simulink model "sampleModel1660"  (R2023a)
settings: Solver=VariableStepAuto  StartTime=0.0  StopTime=10.0  RelTol=1e-3
libraries: hdlsllib x7, simulink x4
settings Model: Creator=user1  LastModifiedBy=user1

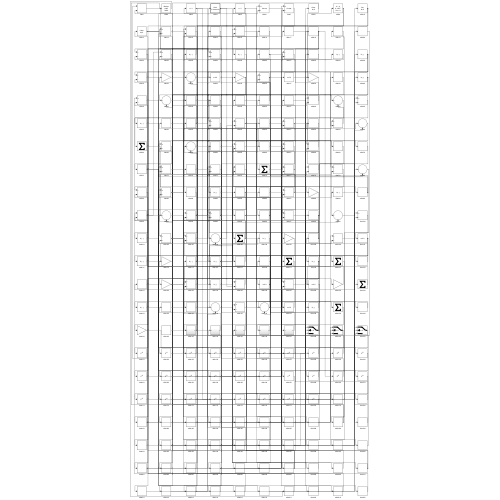
[thumbnail: Simulink's stored preview of the top-level diagram]
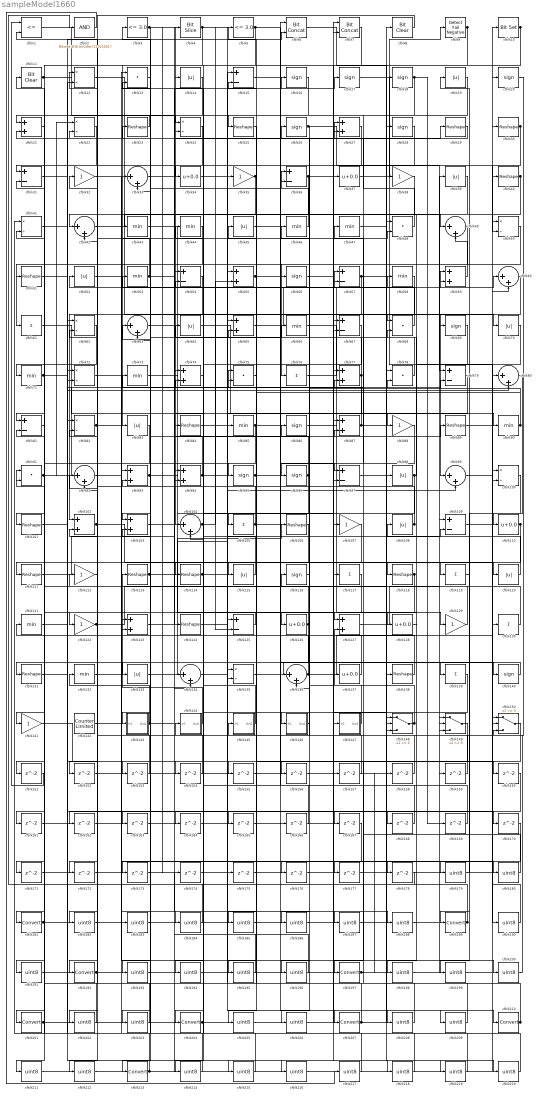
== system sampleModel1660 ==
  cfblk1 : RelationalOperator  Operator=<=  OutDataTypeStr=boolean  InputSameDT=off
  cfblk10 : simulink/Logic and Bit Operations/Bit Set  iBit=0
      settings: LibrarySourceBlock=|
      | hdlsllib/Logic and Bit
      | Operations/Bit Set
  cfblk{12,22,24,41,50,62,72,82,100,135} (10 alike) : Product  Inputs=*/  RndMeth=Zero  SaturateOnIntegerOverflow=on
  cfblk{23,25,29..30,40,51,84,89,101,106,111,113..114,118,124,131,138} (17 alike) : Reshape
  cfblk{21,27,55,59,65,74,77,87,93..94,102..103,123,127} (14 alike) : Sum
  cfblk{33,42,49,60,63,80,92,99,104,134,136} (11 alike) : Sum  Inputs=|++
  cfblk{61,76,105,117,119,130,139} (7 alike) : Sum  Inputs=+
  cfblk{32,35,38,88,107,112,122,129,141} (9 alike) : Gain
  cfblk{14,19,39,45,52,64,70,83,98,108,115,120,133} (13 alike) : Abs  SaturateOnIntegerOverflow=off
  cfblk{15,31,36,54,57,67,79,81,97,109,125} (11 alike) : Sum  Inputs=+-
  cfblk11 : simulink/Logic and Bit Operations/Bit Clear  iBit=0
      settings: LibrarySourceBlock=|
      | hdlsllib/Logic and Bit
      | Operations/Bit Clear
  cfblk{34,37,110,126,128,137} (6 alike) : Bias  Bias=0.0  SaturateOnIntegerOverflow=off
  cfblk{16..18,20,26,28,56,69,86,95..96,116,140} (13 alike) : Signum
  cfblk{43..44,46..47,53,58,66,71,73,85,90,121,132} (13 alike) : MinMax
  cfblk{13,48,68,75,78,91} (6 alike) : DotProduct  OutDataTypeStr=Inherit: Inherit via internal rule
  cfblk142 : hdlsllib/Sources/Counter Limited  uplimit=7  tsamp=-1
  cfblk143 : Subsystem
      settings: LibrarySourceBlock=|
      | hdlsllib/Ports &
      | Subsystems/Subsystem
  cfblk144 : Subsystem
      settings: LibrarySourceBlock=|
      | hdlsllib/Ports &
      | Subsystems/Subsystem
  cfblk145 : Subsystem
      settings: LibrarySourceBlock=|
      | hdlsllib/Ports &
      | Subsystems/Subsystem
  cfblk146 : Subsystem
      settings: LibrarySourceBlock=|
      | hdlsllib/Ports &
      | Subsystems/Subsystem
  cfblk147 : Subsystem
      settings: LibrarySourceBlock=|
      | hdlsllib/Ports &
      | Subsystems/Subsystem
  cfblk148 : Switch  SaturateOnIntegerOverflow=off  InputSameDT=off
  cfblk149 : Switch  SaturateOnIntegerOverflow=off  InputSameDT=off
  cfblk150 : Switch  SaturateOnIntegerOverflow=off  InputSameDT=off
  cfblk{151..178} (28 alike) : Delay  SampleTime=1
  cfblk{179..180,182..188,190..191,193..196,198..200,202..203,205..206,208..209,211..212,214..220} (33 alike) : DataTypeConversion  OutDataTypeStr=uint8  SaturateOnIntegerOverflow=off  RndMeth=Floor
  cfblk{181,189,192,197,201,204,207,210,213} (9 alike) : DataTypeConversion  SaturateOnIntegerOverflow=off  RndMeth=Floor
  cfblk2 : simulink/Logic and Bit Operations/Bitwise Operator  logicop=AND  UseBitMask=on  BitMask=bin2dec('11011001')  BitMaskRealWorld=Stored Integer
      settings: LibrarySourceBlock=|
      | hdlsllib/Logic and Bit
      | Operations/Bitwise
      | Operator
  cfblk3 : hdlsllib/Logic and Bit Operations/Compare To Constant  relop=<=  const=3.0  OutDataTypeStr=boolean
  cfblk4 : hdlsllib/Logic and Bit Operations/Bit Slice  lidx=7  ridx=0
  cfblk5 : hdlsllib/Logic and Bit Operations/Compare To Constant  relop=<=  const=3.0  OutDataTypeStr=boolean
  cfblk6 : hdlsllib/Logic and Bit Operations/Bit Concat  numInputs=2
  cfblk7 : hdlsllib/Logic and Bit Operations/Bit Concat  numInputs=2
  cfblk8 : simulink/Logic and Bit Operations/Bit Clear  iBit=0
      settings: LibrarySourceBlock=|
      | hdlsllib/Logic and Bit
      | Operations/Bit Clear
  cfblk9 : hdlsllib/Logic and Bit Operations/Detect Fall Negative  vinit=0  OutDataTypeStr=boolean
  wires:
  cfblk140/1 -> cfblk131/1
  cfblk123/1 -> cfblk116/1
  cfblk17/1 -> cfblk70/1
  cfblk43/1 -> cfblk126/1
  cfblk102/1 -> cfblk115/1, cfblk48/2, cfblk59/1
  cfblk63/1 -> cfblk127/1
  cfblk88/1 -> cfblk146/1(In1)
  cfblk4/1 -> cfblk83/1, cfblk125/2, cfblk68/1
  cfblk8/1 -> cfblk42/1
  cfblk133/1 -> cfblk106/1
  cfblk49/1 -> cfblk61/1
  cfblk66/1 -> cfblk129/1
  cfblk148/1 -> cfblk127/2, cfblk123/2
  cfblk38/1 -> cfblk104/1
  cfblk135/1 -> cfblk139/1
  cfblk94/1 -> cfblk63/1, cfblk114/1, cfblk89/1
  cfblk12/1 -> cfblk99/1
  cfblk3/1 -> cfblk124/1, cfblk173/1, cfblk174/1
  cfblk5/1 -> cfblk51/1, cfblk180/1
  cfblk103/1 -> cfblk57/1
  cfblk24/1 -> cfblk81/1
  cfblk60/1 -> cfblk102/1
  cfblk145/1(Out1) -> cfblk73/1
  cfblk16/1 -> cfblk42/2
  cfblk42/1 -> cfblk49/1
  cfblk99/1 -> cfblk20/1
  cfblk26/1 -> cfblk79/1, cfblk206/1
  cfblk50/1 -> cfblk76/1
  cfblk14/1 -> cfblk101/1
  cfblk61/1 -> cfblk90/1
  cfblk59/1 -> cfblk49/2
  cfblk90/1 -> cfblk46/1, cfblk65/2
  cfblk118/1 -> cfblk141/1, cfblk211/1
  cfblk46/1 -> cfblk23/1
  cfblk37/1 -> cfblk9/1
  cfblk33/1 -> cfblk4/1
  cfblk11/1 -> cfblk24/1, cfblk6/2, cfblk215/1
  cfblk136/1 -> cfblk40/1, cfblk103/2
  cfblk82/1 -> cfblk16/1, cfblk177/1
  cfblk144/1(Out1) -> cfblk113/1
  cfblk67/1 -> cfblk204/1
  cfblk91/1 -> cfblk79/2, cfblk22/1
  cfblk111/1 -> cfblk29/1
  cfblk86/1 -> cfblk118/1
  cfblk1/1 -> cfblk24/2
  cfblk20/1 -> cfblk145/1(In1)
  cfblk23/1 -> cfblk21/1
  cfblk58/1 -> cfblk143/1(In1)
  cfblk48/1 -> cfblk27/1
  cfblk143/1(Out1) -> cfblk92/1, cfblk66/1
  cfblk127/1 -> cfblk39/1
  cfblk68/1 -> cfblk3/1
  cfblk124/1 -> cfblk35/1
  cfblk57/1 -> cfblk130/1, cfblk162/1
  cfblk73/1 -> cfblk88/1
  cfblk120/1 -> cfblk108/1
  cfblk104/1 -> cfblk14/1, cfblk55/2
  cfblk10/1 -> cfblk57/2, cfblk163/1
  cfblk83/1 -> cfblk111/1
  cfblk72/1 -> cfblk43/1
  cfblk19/1 -> cfblk31/1
  cfblk78/1 -> cfblk36/1
  cfblk138/1 -> cfblk26/1
  cfblk117/1 -> cfblk192/1
  cfblk77/1 -> cfblk52/1, cfblk135/2
  cfblk107/1 -> cfblk181/1
  cfblk76/1 -> cfblk60/1
  cfblk29/1 -> cfblk21/2
  cfblk28/1 -> cfblk54/1
  cfblk98/1 -> cfblk104/2, cfblk136/2, cfblk68/2
  cfblk125/1 -> cfblk122/1
  cfblk80/1 -> cfblk110/1
  cfblk93/1 -> cfblk137/1, cfblk87/2
  cfblk89/1 -> cfblk80/1
  cfblk96/1 -> cfblk105/1, cfblk44/1
  cfblk130/1 -> cfblk91/1
  cfblk122/1 -> cfblk28/1, cfblk200/1
  cfblk142/1 -> cfblk123/1
  cfblk113/1 -> cfblk85/1, cfblk63/2
  cfblk27/1 -> cfblk133/1
  cfblk35/1 -> cfblk92/2, cfblk172/1
  cfblk51/1 -> cfblk80/2
  cfblk64/1 -> cfblk147/1(In1)
  cfblk53/1 -> cfblk17/1, cfblk22/2
  cfblk150/1 -> cfblk197/1
  cfblk114/1 -> cfblk99/2, cfblk109/2
  cfblk6/1 -> cfblk138/1
  cfblk45/1 -> cfblk69/1
  cfblk25/1 -> cfblk95/1
  cfblk13/1 -> cfblk213/1
  cfblk87/1 -> cfblk64/1, cfblk220/1
  cfblk112/1 -> cfblk32/1
  cfblk115/1 -> cfblk93/2
  cfblk40/1 -> cfblk128/1, cfblk182/1
  cfblk7/1 -> cfblk84/1
  cfblk21/1 -> cfblk71/1
  cfblk95/1 -> cfblk56/1, cfblk140/1
  cfblk105/1 -> cfblk136/1, cfblk82/2, cfblk1/2
  cfblk9/1 -> cfblk33/1, cfblk94/2
  cfblk18/1 -> cfblk25/1, cfblk72/2, cfblk97/1, cfblk169/1
  cfblk131/1 -> cfblk75/1
  cfblk146/1(Out1) -> cfblk86/1
  cfblk55/1 -> cfblk119/1, cfblk97/2
  cfblk36/1 -> cfblk148/3, cfblk94/1
  cfblk134/1 -> cfblk210/1
  cfblk108/1 -> cfblk12/1, cfblk45/1
  cfblk62/1 -> cfblk201/1
  cfblk110/1 -> cfblk193/1, cfblk196/1
  cfblk100/1 -> cfblk189/1
  cfblk15/1 -> cfblk207/1
  cfblk85/1 -> cfblk78/2, cfblk103/1
  cfblk126/1 -> cfblk31/2, cfblk165/1
  cfblk129/1 -> cfblk11/1
  cfblk137/1 -> cfblk81/2
  cfblk30/1 -> cfblk50/2, cfblk96/1, cfblk59/2
  cfblk65/1 -> cfblk58/1
  cfblk97/1 -> cfblk120/1
  cfblk71/1 -> cfblk153/1, cfblk154/1
  cfblk147/1(Out1) -> cfblk53/1
  cfblk81/1 -> cfblk151/1
  cfblk151/1 -> cfblk1/1
  cfblk39/1 -> cfblk152/1
  cfblk152/1 -> cfblk78/1
  cfblk153/1 -> cfblk102/2
  cfblk154/1 -> cfblk33/2
  cfblk92/1 -> cfblk155/1
  cfblk155/1 -> cfblk148/1
  cfblk79/1 -> cfblk156/1
  cfblk157/1 -> cfblk93/1
  cfblk158/1 -> cfblk65/1
  cfblk159/1 -> cfblk36/2
  cfblk52/1 -> cfblk160/1
  cfblk22/1 -> cfblk161/1
  cfblk161/1 -> cfblk135/1
  cfblk162/1 -> cfblk87/1
  cfblk163/1 -> cfblk7/2
  cfblk31/1 -> cfblk164/1
  cfblk164/1 -> cfblk77/1
  cfblk141/1 -> cfblk166/1
  cfblk166/1 -> cfblk6/1
  cfblk101/1 -> cfblk167/1
  cfblk128/1 -> cfblk168/1
  cfblk168/1 -> cfblk148/2
  cfblk169/1 -> cfblk54/2
  cfblk56/1 -> cfblk170/1
  cfblk106/1 -> cfblk171/1
  cfblk171/1 -> cfblk27/2
  cfblk172/1 -> cfblk125/1
  cfblk175/1 -> cfblk60/2
  cfblk34/1 -> cfblk176/1
  cfblk176/1 -> cfblk50/1
  cfblk177/1 -> cfblk109/1
  cfblk70/1 -> cfblk178/1
  cfblk178/1 -> cfblk2/1
  cfblk47/1 -> cfblk179/1
  cfblk179/1 -> cfblk19/1
  cfblk180/1 -> cfblk47/1
  cfblk181/1 -> cfblk12/2, cfblk18/1
  cfblk182/1 -> cfblk107/1
  cfblk132/1 -> cfblk183/1
  cfblk183/1 -> cfblk98/1
  cfblk32/1 -> cfblk184/1
  cfblk184/1 -> cfblk132/1
  cfblk149/1 -> cfblk185/1
  cfblk185/1 -> cfblk37/1
  cfblk116/1 -> cfblk186/1
  cfblk186/1 -> cfblk149/1
  cfblk173/1 -> cfblk187/1
  cfblk187/1 -> cfblk149/2
  cfblk165/1 -> cfblk188/1
  cfblk188/1 -> cfblk149/3
  cfblk189/1 -> cfblk82/1, cfblk75/2
  cfblk109/1 -> cfblk190/1
  cfblk190/1 -> cfblk100/1
  cfblk44/1 -> cfblk191/1
  cfblk191/1 -> cfblk100/2
  cfblk192/1 -> cfblk175/1, cfblk38/1
  cfblk193/1 -> cfblk117/1
  cfblk74/1 -> cfblk194/1
  cfblk194/1 -> cfblk48/1
  cfblk75/1 -> cfblk195/1
  cfblk195/1 -> cfblk74/1
  cfblk196/1 -> cfblk74/2
  cfblk197/1 -> cfblk159/1, cfblk158/1
  cfblk69/1 -> cfblk198/1
  cfblk198/1 -> cfblk150/1
  cfblk119/1 -> cfblk199/1
  cfblk199/1 -> cfblk150/2
  cfblk200/1 -> cfblk150/3
  cfblk201/1 -> cfblk34/1, cfblk8/1
  cfblk54/1 -> cfblk202/1
  cfblk202/1 -> cfblk62/1
  cfblk170/1 -> cfblk203/1
  cfblk203/1 -> cfblk62/2
  cfblk204/1 -> cfblk157/1, cfblk7/1
  cfblk167/1 -> cfblk205/1
  cfblk205/1 -> cfblk67/1
  cfblk206/1 -> cfblk67/2
  cfblk207/1 -> cfblk5/1, cfblk112/1, cfblk55/1
  cfblk84/1 -> cfblk208/1
  cfblk208/1 -> cfblk15/1
  cfblk174/1 -> cfblk209/1
  cfblk209/1 -> cfblk15/2
  cfblk210/1 -> cfblk91/2, cfblk77/2
  cfblk211/1 -> cfblk134/1
  cfblk160/1 -> cfblk212/1
  cfblk212/1 -> cfblk134/2
  cfblk213/1 -> cfblk72/1, cfblk10/1
  cfblk139/1 -> cfblk214/1
  cfblk214/1 -> cfblk13/1
  cfblk215/1 -> cfblk13/2
  cfblk121/1 -> cfblk216/1
  cfblk216/1 -> cfblk30/1
  cfblk2/1 -> cfblk217/1
  cfblk217/1 -> cfblk121/1
  cfblk41/1 -> cfblk218/1
  cfblk218/1 -> cfblk144/1(In1)
  cfblk156/1 -> cfblk219/1
  cfblk219/1 -> cfblk41/1
  cfblk220/1 -> cfblk41/2

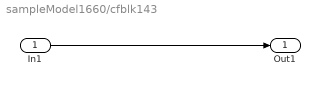
== system sampleModel1660/cfblk143 ==
  In1 : Inport
  Out1 : Outport
  wires:
  In1/1 -> Out1/1

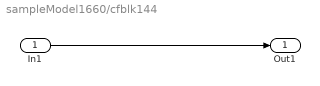
== system sampleModel1660/cfblk144 ==
  In1 : Inport
  Out1 : Outport
  wires:
  In1/1 -> Out1/1

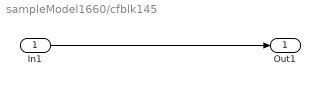
== system sampleModel1660/cfblk145 ==
  In1 : Inport
  Out1 : Outport
  wires:
  In1/1 -> Out1/1

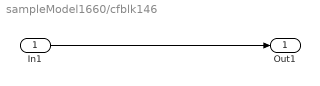
== system sampleModel1660/cfblk146 ==
  In1 : Inport
  Out1 : Outport
  wires:
  In1/1 -> Out1/1

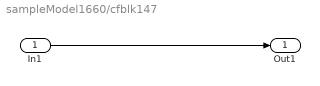
== system sampleModel1660/cfblk147 ==
  In1 : Inport
  Out1 : Outport
  wires:
  In1/1 -> Out1/1
